simulink model "exampleModel_bus_axi_w_4ptavg"  (R2017b)
settings: Solver=VariableStepAuto  StartTime=0.0  StopTime=10e-5  RelTol=1e-3
PreLoadFcn:
  | setup
values from neighbouring files (symbols this model uses):
  axiClk = 156.25e6    (= 156250000)    [setup.m]    (also in setup_exampleModel_bus_axi_simulink.m; setup_exampleModel_bus_axi_simulink_lcls2.m; setup_lcls2_pcav.m; sysgen_signal.m)
  cav1p1_addr = 204    [setup_exampleModel_bus_axi_simulink.m]    (also in setup_exampleModel_bus_axi_simulink_lcls2.m; setup_lcls2_pcav.m; sysgen_signal.m)
  cav1p2_addr = cav1p1_addr * 2    (= 408)    [setup_exampleModel_bus_axi_simulink.m]    (also in setup_exampleModel_bus_axi_simulink_lcls2.m; setup_lcls2_pcav.m; sysgen_signal.m)
  cav2p1_addr = cav1p1_addr * 3    (= 612)    [setup_exampleModel_bus_axi_simulink.m]    (also in setup_exampleModel_bus_axi_simulink_lcls2.m; setup_lcls2_pcav.m; sysgen_signal.m)
  cav2p2_addr = cav1p1_addr * 4    (= 816)    [setup_exampleModel_bus_axi_simulink.m]    (also in setup_exampleModel_bus_axi_simulink_lcls2.m; setup_lcls2_pcav.m; sysgen_signal.m)
  Fadc = Fs/interleavedChannels    (= 29750000)    [setup.m]    (also in setup_exampleModel_bus_axi_simulink.m = 357000000; setup_exampleModel_bus_axi_simulink_lcls2.m = 351000000; setup_lcls2_pcav.m = 357000000; sysgen_signal.m = 357000000)
  fir_lpf = fir1(15, w_lpf)    [setup_exampleModel_bus_axi_simulink.m]    (also in setup_exampleModel_bus_axi_simulink_lcls2.m; setup_lcls2_pcav.m)
  Fproc = 204e6    (= 204000000)    [setup_exampleModel_bus_axi_simulink.m]    (also in setup_exampleModel_bus_axi_simulink_lcls2.m = 200571400; setup_lcls2_pcav.m; sysgen_signal.m)
  Fsig = Fproc/12    (= 17000000)    [setup_exampleModel_bus_axi_simulink.m]    (also in setup_exampleModel_bus_axi_simulink_lcls2.m = 16714283.3333; setup_lcls2_pcav.m)
  Tadc = 1/fadc    (= 2.80112044818e-09)    [cavity_signal.m]    (also in setup_exampleModel_bus_axi_simulink.m; setup_exampleModel_bus_axi_simulink_lcls2.m = 2.849002849e-09; setup_lcls2_pcav.m; setup_pcav_simulink.m)
undefined symbols (not defined in the file or in its folder): AXI4, Lite
libraries: xbsIndex_r4 x2870, llrf_lib x10, simulink x3
(part 14 of 15)

== system exampleModel_bus_axi_w_4ptavg/example/dsp/Cav2/Subsystem2/freq_err1/delta_phi ==
  note: 3.14
  note: calculating delta phi
  note: d(scaled_phi)
  phase : Inport
  window : Inport  Port=2
  reset : Inport  Port=3
  AddSub3 : xbsIndex_r4/AddSub  mode=Subtraction  use_carryin=off  use_carryout=off  en=on  latency=1  precision=Full  arith_type="Signed  (2's comp)"  n_bits=32  bin_pt=30  quantization=Truncate  overflow=Saturate  use_behavioral_HDL=off  hw_selection=Fabric  pipelined=off  dbl_ovrd=off  block_type=addsub
  Constant : xbsIndex_r4/Constant  const=0  gui_display_data_type=Fixed-point  arith_type=Signed (2's comp)  n_bits=1  bin_pt=0  preci_type=Single  exp_width=8  frac_width=24  explicit_period=off  period=1  equ=P=C  opselect=C  inp2=PCIN>>17  opr=+  inp1=P  carry=CIN  dbl_ovrd=off  block_type=constant
  Constant1 : xbsIndex_r4/Constant  const=0  gui_display_data_type=Fixed-point  arith_type=Signed (2's comp)  n_bits=1  bin_pt=0  preci_type=Single  exp_width=8  frac_width=24  explicit_period=off  period=1  equ=P=C  opselect=C  inp2=PCIN>>17  opr=+  inp1=P  carry=CIN  dbl_ovrd=off  block_type=constant
  Constant4 : xbsIndex_r4/Constant  const=pi  gui_display_data_type=Fixed-point  arith_type=Signed (2's comp)  n_bits=18  bin_pt=15  preci_type=Single  exp_width=8  frac_width=24  explicit_period=off  period=1  equ=P=C  opselect=C  inp2=PCIN>>17  opr=+  inp1=P  carry=CIN  dbl_ovrd=off  block_type=constant
  Convert1 : xbsIndex_r4/Convert  gui_display_data_type=Boolean  arith_type=Boolean  n_bits=16  bin_pt=14  float_type=Single  exp_bits=8  fraction_bits=24  quantization=Truncate  overflow=Wrap  en=off  latency=1  pipeline=off  dbl_ovrd=off  block_type=convert
  Delay2 : xbsIndex_r4/Delay  rst=off  infoeditControl=Selection of Reset will increase slice count due to use of real FFs and instead of SRLs  en=off  latency=2  reg_retiming=off  dbl_ovrd=off  block_type=delay
  Display{,1..2,5} (4 alike) : Display
  Gateway Out{3,27..29} (4 alike) : xbsIndex_r4/Gateway Out  inherit_from_input=off  hdl_port=on  rows=1  columns=1  UseAsDAC=off  DACChannel='1'  interface=None  automatic_assignment=on  address_offset=hex2dec('00')  intf_name=''  intf_description=''  timing_constraint=None  locs_specified=off  LOCs={}  io_standard={}  block_type=gatewayout
  Inverter : xbsIndex_r4/Inverter  en=off  latency=1  dbl_ovrd=off  block_type=inv
  Logical : xbsIndex_r4/Logical  logical_function=AND  inputs=2  en=off  latency=1  precision=User Defined  arith_type=Boolean  n_bits=1  bin_pt=0  align_bp=on  dbl_ovrd=off  block_type=logical
  Mult1 : xbsIndex_r4/Mult  precision=User Defined  arith_type="Signed  (2's comp)"  n_bits=32  bin_pt=30  quantization=Truncate  overflow=Saturate  en=off  latency=3  use_behavioral_HDL=off  opt=Speed  use_embedded=on  optimum_pipeline=off  pipeline=on  dbl_ovrd=off  use_rpm=on  placement_style=Triangular  block_type=mult
  Relational : xbsIndex_r4/Relational  mode=a!=b  op_type=Bool  en=off  latency=1  dbl_ovrd=off  block_type=relational
  Relational1 : xbsIndex_r4/Relational  mode=a!=b  op_type=Bool  en=off  latency=1  dbl_ovrd=off  block_type=relational
  low_bit : Scope  NumInputPorts=4
  phase_latching : Subsystem
  d_phi : Outport
  val_latched : Outport  Port=2
  wires:
  Logical/1 -> val_latched/1
  Relational1/1 -> Logical/2
  Relational/1 -> Logical/1
  phase_latching/2(Start_value) -> AddSub3/2, Gateway Out28/1, Relational1/1
  Constant1/1 -> Relational1/2
  Constant/1 -> Relational/2
  phase_latching/1(Stop_value) -> Gateway Out29/1, Relational/1, AddSub3/1
  window/1 -> phase_latching/2(window), Convert1/1
  Convert1/1 -> Inverter/1
  Gateway Out27/1 -> Display2/1, low_bit/3
  Gateway Out28/1 -> Display1/1, low_bit/2
  AddSub3/1 -> Gateway Out27/1, Mult1/1
  phase/1 -> phase_latching/1(phase)
  Mult1/1 -> Gateway Out3/1, d_phi/1
  Gateway Out29/1 -> Display/1, low_bit/1
  Delay2/1 -> AddSub3/3
  Gateway Out3/1 -> Display5/1, low_bit/4
  Constant4/1 -> Mult1/2
  Inverter/1 -> Delay2/1
  reset/1 -> phase_latching/3(reset)

== system exampleModel_bus_axi_w_4ptavg/example/dsp/Cav2/Subsystem2/freq_err1/delta_t ==
  note: (2*pi)/(Fsig)
  window : Inport
  reset : Inport  Port=2
  Constant5 : xbsIndex_r4/Constant  const=(2*pi)/(Fsig)  gui_display_data_type=Fixed-point  arith_type=Unsigned  n_bits=32  bin_pt=32  preci_type=Single  exp_width=8  frac_width=24  explicit_period=off  period=1  equ=P=C  opselect=C  inp2=PCIN>>17  opr=+  inp1=P  carry=CIN  dbl_ovrd=off  block_type=constant
  Convert1 : xbsIndex_r4/Convert  gui_display_data_type=Boolean  arith_type=Boolean  n_bits=16  bin_pt=14  float_type=Single  exp_bits=8  fraction_bits=24  quantization=Truncate  overflow=Wrap  en=off  latency=1  pipeline=off  dbl_ovrd=off  block_type=convert
  Counter2 : xbsIndex_r4/Counter  cnt_type=Free Running  cnt_to=Inf  operation=Up  start_count=0  cnt_by_val=1  arith_type=Unsigned  n_bits=10  bin_pt=0  load_pin=off  rst=on  en=on  explicit_period=on  period=1/(17e6)  use_behavioral_HDL=off  implementation=Fabric  dbl_ovrd=off  block_type=counter
  Display3 : Display
  Display4 : Display
  Gateway Out1 : xbsIndex_r4/Gateway Out  inherit_from_input=off  hdl_port=on  rows=1  columns=1  UseAsDAC=off  DACChannel='1'  interface=None  automatic_assignment=on  address_offset=hex2dec('00')  intf_name=''  intf_description=''  timing_constraint=None  locs_specified=off  LOCs={}  io_standard={}  block_type=gatewayout
  Gateway Out2 : xbsIndex_r4/Gateway Out  inherit_from_input=off  hdl_port=on  rows=1  columns=1  UseAsDAC=off  DACChannel='1'  interface=None  automatic_assignment=on  address_offset=hex2dec('00')  intf_name=''  intf_description=''  timing_constraint=None  locs_specified=off  LOCs={}  io_standard={}  block_type=gatewayout
  Inverter : xbsIndex_r4/Inverter  en=off  latency=1  dbl_ovrd=off  block_type=inv
  Mult : xbsIndex_r4/Mult  precision=User Defined  arith_type="Signed  (2's comp)"  n_bits=32  bin_pt=32  quantization=Truncate  overflow=Saturate  en=off  latency=3  use_behavioral_HDL=off  opt=Speed  use_embedded=on  optimum_pipeline=off  pipeline=on  dbl_ovrd=off  use_rpm=on  placement_style=Triangular  block_type=mult
  Register2 : xbsIndex_r4/Register  init=0  rst=on  en=on  dbl_ovrd=off  block_type=register
  dt : Outport
  wires:
  Gateway Out1/1 -> Display3/1
  window/1 -> Convert1/1
  Mult/1 -> Gateway Out1/1, dt/1
  Constant5/1 -> Mult/2
  Convert1/1 -> Counter2/2, Inverter/1
  Inverter/1 -> Register2/3
  Counter2/1 -> Register2/1
  Gateway Out2/1 -> Display4/1
  Register2/1 -> Gateway Out2/1, Mult/1
  reset/1 -> Counter2/1, Register2/2

== system exampleModel_bus_axi_w_4ptavg/example/dsp/Cav2/Subsystem4/freq_err1/Subsystem ==
  In1 : Inport
  In2 : Inport  Port=2
  AddSub : xbsIndex_r4/AddSub  mode=Addition  use_carryin=off  use_carryout=off  en=on  latency=1  precision=User Defined  arith_type="Signed  (2's comp)"  n_bits=64  bin_pt=32  quantization=Truncate  overflow=Saturate  use_behavioral_HDL=off  hw_selection=Fabric  pipelined=off  dbl_ovrd=off  block_type=addsub
  Constant1 : xbsIndex_r4/Constant  const=-Fsig  gui_display_data_type=Fixed-point  arith_type=Signed (2's comp)  n_bits=26  bin_pt=0  preci_type=Single  exp_width=8  frac_width=24  explicit_period=off  period=1  equ=P=C  opselect=C  inp2=PCIN>>17  opr=+  inp1=P  carry=CIN  dbl_ovrd=off  block_type=constant
  Convert1 : xbsIndex_r4/Convert  gui_display_data_type=Fixed-point  arith_type="Signed  (2's comp)"  n_bits=32  bin_pt=32  float_type=Single  exp_bits=8  fraction_bits=24  quantization=Truncate  overflow=Saturate  en=off  latency=1  pipeline=off  dbl_ovrd=off  block_type=convert
  Delay3 : xbsIndex_r4/Delay  rst=off  infoeditControl=Selection of Reset will increase slice count due to use of real FFs and instead of SRLs  en=off  latency=10  reg_retiming=off  dbl_ovrd=off  block_type=delay
  Delay4 : xbsIndex_r4/Delay  rst=off  infoeditControl=Selection of Reset will increase slice count due to use of real FFs and instead of SRLs  en=off  latency=1  reg_retiming=off  dbl_ovrd=off  block_type=delay
  Delay5 : xbsIndex_r4/Delay  rst=off  infoeditControl=Selection of Reset will increase slice count due to use of real FFs and instead of SRLs  en=off  latency=1  reg_retiming=off  dbl_ovrd=off  block_type=delay
  Display1 : Display
  Divide2 : xbsIndex_r4/Divide  flow_control=NonBlocking  axi_optimize_goal=Resources  algorithm_type=Radix2  infoedit1=Specify output fraction-width for Fixed-point division.  fractional_width=33  infoedit2=Specify latency for Floating-point division.  latency=1  rate=1  has_a_tlast=off  has_a_tuser=off  has_b_tlast=off  has_b_tuser=off  en=off  has_result_tready=off  result_tlast_behv=Pass_A_TLAST  has_underflow=off  has_overflow=off  has_invalid_op=off  has_divide_by_zero=off  fpo_op_type=mergeddivide  block_type=divide
      settings: infoedit=Blocking: Wait for data on all inputs, allow back-pressure.<br>NonBlocking: operate every cycle in which all inputs are valid, no back-pressure.
  Down Sample1 : xbsIndex_r4/Down Sample  sample_ratio=12  sample_phase="Last Value of Frame  (most efficient)"  en=off  rst=off  latency=1  dbl_ovrd=off  block_type=dsamp
  Down Sample8 : xbsIndex_r4/Down Sample  sample_ratio=12  sample_phase="Last Value of Frame  (most efficient)"  en=off  rst=off  latency=1  dbl_ovrd=off  block_type=dsamp
  Gateway Out{5..7,9} (4 alike) : xbsIndex_r4/Gateway Out  inherit_from_input=off  hdl_port=on  rows=1  columns=1  UseAsDAC=off  DACChannel='1'  interface=None  automatic_assignment=on  address_offset=hex2dec('00')  intf_name=''  intf_description=''  timing_constraint=None  locs_specified=off  LOCs={}  io_standard={}  block_type=gatewayout
  Inverter : xbsIndex_r4/Inverter  en=off  latency=1  dbl_ovrd=off  block_type=inv
  Logical1 : xbsIndex_r4/Logical  logical_function=AND  inputs=2  en=off  latency=1  precision=User Defined  arith_type=Boolean  n_bits=1  bin_pt=0  align_bp=on  dbl_ovrd=off  block_type=logical
  Register : xbsIndex_r4/Register  init=0  rst=on  en=on  dbl_ovrd=off  block_type=register
  Scope3 : Scope  NumInputPorts=3
  Scope4 : Scope  NumInputPorts=3
  tag scope: testb=global
  wires:
  Delay3/1 -> Logical1/2, Inverter/1
  Logical1/1 -> Gateway Out6/1, Delay4/1, Delay5/1, Register/3
  Constant1/1 -> Divide2/2
  Inverter/1 -> Logical1/1
  Divide2/1 -> Down Sample1/1
  Register/1 -> AddSub/1, Gateway Out5/1
  Gateway Out5/1 -> Scope3/2
  In2/1 -> Down Sample8/1
  Convert1/1 -> [testb]
  Down Sample8/1 -> Register/1
  Delay5/1 -> Register/2
  Delay4/1 -> AddSub/3
  Gateway Out6/1 -> Scope3/3
  In1/1 -> Delay3/1
  AddSub/1 -> AddSub/2, Gateway Out7/1, Divide2/1, Gateway Out9/1
  Down Sample1/1 -> Convert1/1
  Gateway Out7/1 -> Scope3/1, Display1/1
  Gateway Out9/1 -> Scope4/1

== system exampleModel_bus_axi_w_4ptavg/example/dsp/Cav2/Subsystem4/freq_err1/delta_phi ==
  note: 3.14
  note: calculating delta phi
  note: d(scaled_phi)
  phase : Inport
  window : Inport  Port=2
  reset : Inport  Port=3
  AddSub3 : xbsIndex_r4/AddSub  mode=Subtraction  use_carryin=off  use_carryout=off  en=on  latency=1  precision=Full  arith_type="Signed  (2's comp)"  n_bits=32  bin_pt=30  quantization=Truncate  overflow=Saturate  use_behavioral_HDL=off  hw_selection=Fabric  pipelined=off  dbl_ovrd=off  block_type=addsub
  Constant : xbsIndex_r4/Constant  const=0  gui_display_data_type=Fixed-point  arith_type=Signed (2's comp)  n_bits=1  bin_pt=0  preci_type=Single  exp_width=8  frac_width=24  explicit_period=off  period=1  equ=P=C  opselect=C  inp2=PCIN>>17  opr=+  inp1=P  carry=CIN  dbl_ovrd=off  block_type=constant
  Constant1 : xbsIndex_r4/Constant  const=0  gui_display_data_type=Fixed-point  arith_type=Signed (2's comp)  n_bits=1  bin_pt=0  preci_type=Single  exp_width=8  frac_width=24  explicit_period=off  period=1  equ=P=C  opselect=C  inp2=PCIN>>17  opr=+  inp1=P  carry=CIN  dbl_ovrd=off  block_type=constant
  Constant4 : xbsIndex_r4/Constant  const=pi  gui_display_data_type=Fixed-point  arith_type=Signed (2's comp)  n_bits=18  bin_pt=15  preci_type=Single  exp_width=8  frac_width=24  explicit_period=off  period=1  equ=P=C  opselect=C  inp2=PCIN>>17  opr=+  inp1=P  carry=CIN  dbl_ovrd=off  block_type=constant
  Convert1 : xbsIndex_r4/Convert  gui_display_data_type=Boolean  arith_type=Boolean  n_bits=16  bin_pt=14  float_type=Single  exp_bits=8  fraction_bits=24  quantization=Truncate  overflow=Wrap  en=off  latency=1  pipeline=off  dbl_ovrd=off  block_type=convert
  Delay2 : xbsIndex_r4/Delay  rst=off  infoeditControl=Selection of Reset will increase slice count due to use of real FFs and instead of SRLs  en=off  latency=2  reg_retiming=off  dbl_ovrd=off  block_type=delay
  Display{,1..2,5} (4 alike) : Display
  Gateway Out{3,27..29} (4 alike) : xbsIndex_r4/Gateway Out  inherit_from_input=off  hdl_port=on  rows=1  columns=1  UseAsDAC=off  DACChannel='1'  interface=None  automatic_assignment=on  address_offset=hex2dec('00')  intf_name=''  intf_description=''  timing_constraint=None  locs_specified=off  LOCs={}  io_standard={}  block_type=gatewayout
  Inverter : xbsIndex_r4/Inverter  en=off  latency=1  dbl_ovrd=off  block_type=inv
  Logical : xbsIndex_r4/Logical  logical_function=AND  inputs=2  en=off  latency=1  precision=User Defined  arith_type=Boolean  n_bits=1  bin_pt=0  align_bp=on  dbl_ovrd=off  block_type=logical
  Mult1 : xbsIndex_r4/Mult  precision=User Defined  arith_type="Signed  (2's comp)"  n_bits=32  bin_pt=30  quantization=Truncate  overflow=Saturate  en=off  latency=3  use_behavioral_HDL=off  opt=Speed  use_embedded=on  optimum_pipeline=off  pipeline=on  dbl_ovrd=off  use_rpm=on  placement_style=Triangular  block_type=mult
  Relational : xbsIndex_r4/Relational  mode=a!=b  op_type=Bool  en=off  latency=1  dbl_ovrd=off  block_type=relational
  Relational1 : xbsIndex_r4/Relational  mode=a!=b  op_type=Bool  en=off  latency=1  dbl_ovrd=off  block_type=relational
  low_bit : Scope  NumInputPorts=4
  phase_latching : Subsystem
  d_phi : Outport
  val_latched : Outport  Port=2
  wires:
  Logical/1 -> val_latched/1
  Relational1/1 -> Logical/2
  Relational/1 -> Logical/1
  phase_latching/2(Start_value) -> AddSub3/2, Gateway Out28/1, Relational1/1
  Constant1/1 -> Relational1/2
  Constant/1 -> Relational/2
  phase_latching/1(Stop_value) -> Gateway Out29/1, Relational/1, AddSub3/1
  window/1 -> phase_latching/2(window), Convert1/1
  Convert1/1 -> Inverter/1
  Gateway Out27/1 -> Display2/1, low_bit/3
  Gateway Out28/1 -> Display1/1, low_bit/2
  AddSub3/1 -> Gateway Out27/1, Mult1/1
  phase/1 -> phase_latching/1(phase)
  Mult1/1 -> Gateway Out3/1, d_phi/1
  Gateway Out29/1 -> Display/1, low_bit/1
  Delay2/1 -> AddSub3/3
  Gateway Out3/1 -> Display5/1, low_bit/4
  Constant4/1 -> Mult1/2
  Inverter/1 -> Delay2/1
  reset/1 -> phase_latching/3(reset)

== system exampleModel_bus_axi_w_4ptavg/example/dsp/Cav2/Subsystem4/freq_err1/delta_t ==
  note: (2*pi)/(Fsig)
  window : Inport
  reset : Inport  Port=2
  Constant5 : xbsIndex_r4/Constant  const=(2*pi)/(Fsig)  gui_display_data_type=Fixed-point  arith_type=Unsigned  n_bits=32  bin_pt=32  preci_type=Single  exp_width=8  frac_width=24  explicit_period=off  period=1  equ=P=C  opselect=C  inp2=PCIN>>17  opr=+  inp1=P  carry=CIN  dbl_ovrd=off  block_type=constant
  Convert1 : xbsIndex_r4/Convert  gui_display_data_type=Boolean  arith_type=Boolean  n_bits=16  bin_pt=14  float_type=Single  exp_bits=8  fraction_bits=24  quantization=Truncate  overflow=Wrap  en=off  latency=1  pipeline=off  dbl_ovrd=off  block_type=convert
  Counter2 : xbsIndex_r4/Counter  cnt_type=Free Running  cnt_to=Inf  operation=Up  start_count=0  cnt_by_val=1  arith_type=Unsigned  n_bits=10  bin_pt=0  load_pin=off  rst=on  en=on  explicit_period=on  period=1/(17e6)  use_behavioral_HDL=off  implementation=Fabric  dbl_ovrd=off  block_type=counter
  Display3 : Display
  Display4 : Display
  Gateway Out1 : xbsIndex_r4/Gateway Out  inherit_from_input=off  hdl_port=on  rows=1  columns=1  UseAsDAC=off  DACChannel='1'  interface=None  automatic_assignment=on  address_offset=hex2dec('00')  intf_name=''  intf_description=''  timing_constraint=None  locs_specified=off  LOCs={}  io_standard={}  block_type=gatewayout
  Gateway Out2 : xbsIndex_r4/Gateway Out  inherit_from_input=off  hdl_port=on  rows=1  columns=1  UseAsDAC=off  DACChannel='1'  interface=None  automatic_assignment=on  address_offset=hex2dec('00')  intf_name=''  intf_description=''  timing_constraint=None  locs_specified=off  LOCs={}  io_standard={}  block_type=gatewayout
  Inverter : xbsIndex_r4/Inverter  en=off  latency=1  dbl_ovrd=off  block_type=inv
  Mult : xbsIndex_r4/Mult  precision=User Defined  arith_type="Signed  (2's comp)"  n_bits=32  bin_pt=32  quantization=Truncate  overflow=Saturate  en=off  latency=3  use_behavioral_HDL=off  opt=Speed  use_embedded=on  optimum_pipeline=off  pipeline=on  dbl_ovrd=off  use_rpm=on  placement_style=Triangular  block_type=mult
  Register2 : xbsIndex_r4/Register  init=0  rst=on  en=on  dbl_ovrd=off  block_type=register
  dt : Outport
  wires:
  Gateway Out1/1 -> Display3/1
  window/1 -> Convert1/1
  Mult/1 -> Gateway Out1/1, dt/1
  Constant5/1 -> Mult/2
  Convert1/1 -> Counter2/2, Inverter/1
  Inverter/1 -> Register2/3
  Counter2/1 -> Register2/1
  Gateway Out2/1 -> Display4/1
  Register2/1 -> Gateway Out2/1, Mult/1
  reset/1 -> Counter2/1, Register2/2

== system exampleModel_bus_axi_w_4ptavg/example/dsp/Cav2/c2p1_window_wf /Delay_calc1/Subsystem ==
  In1 : Inport
  Delay3 : xbsIndex_r4/Delay  rst=off  infoeditControl=Selection of Reset will increase slice count due to use of real FFs and instead of SRLs  en=off  latency=2  reg_retiming=off  dbl_ovrd=off  block_type=delay
  Inverter5 : xbsIndex_r4/Inverter  en=off  latency=1  dbl_ovrd=off  block_type=inv
  Logical1 : xbsIndex_r4/Logical  logical_function=AND  inputs=2  en=off  latency=1  precision=Full  arith_type=Unsigned  n_bits=16  bin_pt=0  align_bp=on  dbl_ovrd=off  block_type=logical
  Out1 : Outport
  wires:
  In1/1 -> Inverter5/1, Delay3/1
  Inverter5/1 -> Logical1/1
  Logical1/1 -> Out1/1
  Delay3/1 -> Logical1/2

== system exampleModel_bus_axi_w_4ptavg/example/dsp/Cav2/c2p1_window_wf /Delay_calc1/Subsystem1 ==
  lc : Inport
  d : Inport  Port=2
  qb : Inport  Port=3
  Inverter1 : xbsIndex_r4/Inverter  en=off  latency=1  dbl_ovrd=off  block_type=inv
  Logical6 : xbsIndex_r4/Logical  logical_function=OR  inputs=2  en=off  latency=1  precision=Full  arith_type=Unsigned  n_bits=16  bin_pt=0  align_bp=on  dbl_ovrd=off  block_type=logical
  Register1 : xbsIndex_r4/Register  init=0  rst=off  en=on  dbl_ovrd=off  block_type=register
  q : Outport
  wires:
  qb/1 -> Inverter1/1
  d/1 -> Register1/1
  Logical6/1 -> Register1/2
  lc/1 -> Logical6/2
  Register1/1 -> q/1
  Inverter1/1 -> Logical6/1

== system exampleModel_bus_axi_w_4ptavg/example/dsp/Cav2/c2p1_window_wf /Delay_calc1/Subsystem2 ==
  lc : Inport
  d : Inport  Port=2
  qb : Inport  Port=3
  Inverter1 : xbsIndex_r4/Inverter  en=off  latency=1  dbl_ovrd=off  block_type=inv
  Logical6 : xbsIndex_r4/Logical  logical_function=OR  inputs=2  en=off  latency=1  precision=Full  arith_type=Unsigned  n_bits=16  bin_pt=0  align_bp=on  dbl_ovrd=off  block_type=logical
  Register1 : xbsIndex_r4/Register  init=0  rst=off  en=on  dbl_ovrd=off  block_type=register
  q : Outport
  wires:
  Inverter1/1 -> Logical6/1
  Register1/1 -> q/1
  lc/1 -> Logical6/2
  Logical6/1 -> Register1/2
  d/1 -> Register1/1
  qb/1 -> Inverter1/1

== system exampleModel_bus_axi_w_4ptavg/example/dsp/Cav2/c2p1_window_wf /Delay_calc1/Subsystem3 ==
  In1 : Inport
  In2 : Inport  Port=2
  Gateway Out{1..2,18..19} (4 alike) : xbsIndex_r4/Gateway Out  inherit_from_input=off  hdl_port=off  rows=1  columns=1  UseAsDAC=off  DACChannel='1'  interface=None  automatic_assignment=on  address_offset=hex2dec('00')  intf_name=''  intf_description=''  timing_constraint=None  locs_specified=off  LOCs={}  io_standard={}  block_type=gatewayout
  Logical2 : xbsIndex_r4/Logical  logical_function=AND  inputs=2  en=off  latency=1  precision=Full  arith_type=Unsigned  n_bits=16  bin_pt=0  align_bp=on  dbl_ovrd=off  block_type=logical
  Logical7 : xbsIndex_r4/Logical  logical_function=OR  inputs=2  en=off  latency=1  precision=Full  arith_type=Unsigned  n_bits=16  bin_pt=0  align_bp=on  dbl_ovrd=off  block_type=logical
  Scope1 : Scope  NumInputPorts=2
  Scope3 : Scope  NumInputPorts=2
  and : Outport
  or : Outport  Port=2
  wires:
  In1/1 -> Gateway Out18/1, Logical7/1, Logical2/1
  Logical7/1 -> Gateway Out2/1, or/1
  In2/1 -> Gateway Out19/1, Logical2/2, Logical7/2
  Logical2/1 -> Gateway Out1/1, and/1
  Gateway Out19/1 -> Scope3/2
  Gateway Out18/1 -> Scope3/1
  Gateway Out1/1 -> Scope1/1
  Gateway Out2/1 -> Scope1/2

== system exampleModel_bus_axi_w_4ptavg/example/dsp/Cav2/c2p1_window_wf /Delay_calc1/negedge ==
  d : Inport
  Delay1 : xbsIndex_r4/Delay  rst=off  infoeditControl=Selection of Reset will increase slice count due to use of real FFs and instead of SRLs  en=off  latency=4  reg_retiming=off  dbl_ovrd=off  block_type=delay
  Delay2 : xbsIndex_r4/Delay  rst=off  infoeditControl=Selection of Reset will increase slice count due to use of real FFs and instead of SRLs  en=off  latency=20  reg_retiming=off  dbl_ovrd=off  block_type=delay
  Inverter4 : xbsIndex_r4/Inverter  en=off  latency=1  dbl_ovrd=off  block_type=inv
  Logical7 : xbsIndex_r4/Logical  logical_function=AND  inputs=2  en=off  latency=1  precision=Full  arith_type=Unsigned  n_bits=16  bin_pt=0  align_bp=on  dbl_ovrd=off  block_type=logical
  q : Outport
  wires:
  Delay1/1 -> Logical7/2
  d/1 -> Delay2/1
  Inverter4/1 -> Logical7/1
  Logical7/1 -> q/1
  Delay2/1 -> Inverter4/1, Delay1/1

== system exampleModel_bus_axi_w_4ptavg/example/dsp/Cav2/c2p1_window_wf /Delay_calc2/Subsystem ==
  In1 : Inport
  Delay3 : xbsIndex_r4/Delay  rst=off  infoeditControl=Selection of Reset will increase slice count due to use of real FFs and instead of SRLs  en=off  latency=2  reg_retiming=off  dbl_ovrd=off  block_type=delay
  Inverter5 : xbsIndex_r4/Inverter  en=off  latency=1  dbl_ovrd=off  block_type=inv
  Logical1 : xbsIndex_r4/Logical  logical_function=AND  inputs=2  en=off  latency=1  precision=Full  arith_type=Unsigned  n_bits=16  bin_pt=0  align_bp=on  dbl_ovrd=off  block_type=logical
  Out1 : Outport
  wires:
  In1/1 -> Inverter5/1, Delay3/1
  Inverter5/1 -> Logical1/1
  Logical1/1 -> Out1/1
  Delay3/1 -> Logical1/2

== system exampleModel_bus_axi_w_4ptavg/example/dsp/Cav2/c2p1_window_wf /Delay_calc2/Subsystem1 ==
  lc : Inport
  d : Inport  Port=2
  qb : Inport  Port=3
  Inverter1 : xbsIndex_r4/Inverter  en=off  latency=1  dbl_ovrd=off  block_type=inv
  Logical6 : xbsIndex_r4/Logical  logical_function=OR  inputs=2  en=off  latency=1  precision=Full  arith_type=Unsigned  n_bits=16  bin_pt=0  align_bp=on  dbl_ovrd=off  block_type=logical
  Register1 : xbsIndex_r4/Register  init=0  rst=off  en=on  dbl_ovrd=off  block_type=register
  q : Outport
  wires:
  qb/1 -> Inverter1/1
  d/1 -> Register1/1
  Logical6/1 -> Register1/2
  lc/1 -> Logical6/2
  Register1/1 -> q/1
  Inverter1/1 -> Logical6/1

== system exampleModel_bus_axi_w_4ptavg/example/dsp/Cav2/c2p1_window_wf /Delay_calc2/Subsystem2 ==
  lc : Inport
  d : Inport  Port=2
  qb : Inport  Port=3
  Inverter1 : xbsIndex_r4/Inverter  en=off  latency=1  dbl_ovrd=off  block_type=inv
  Logical6 : xbsIndex_r4/Logical  logical_function=OR  inputs=2  en=off  latency=1  precision=Full  arith_type=Unsigned  n_bits=16  bin_pt=0  align_bp=on  dbl_ovrd=off  block_type=logical
  Register1 : xbsIndex_r4/Register  init=0  rst=off  en=on  dbl_ovrd=off  block_type=register
  q : Outport
  wires:
  Inverter1/1 -> Logical6/1
  Register1/1 -> q/1
  lc/1 -> Logical6/2
  Logical6/1 -> Register1/2
  d/1 -> Register1/1
  qb/1 -> Inverter1/1

== system exampleModel_bus_axi_w_4ptavg/example/dsp/Cav2/c2p1_window_wf /Delay_calc2/Subsystem3 ==
  In1 : Inport
  In2 : Inport  Port=2
  Gateway Out{1..2,18..19} (4 alike) : xbsIndex_r4/Gateway Out  inherit_from_input=off  hdl_port=off  rows=1  columns=1  UseAsDAC=off  DACChannel='1'  interface=None  automatic_assignment=on  address_offset=hex2dec('00')  intf_name=''  intf_description=''  timing_constraint=None  locs_specified=off  LOCs={}  io_standard={}  block_type=gatewayout
  Logical2 : xbsIndex_r4/Logical  logical_function=AND  inputs=2  en=off  latency=1  precision=Full  arith_type=Unsigned  n_bits=16  bin_pt=0  align_bp=on  dbl_ovrd=off  block_type=logical
  Logical7 : xbsIndex_r4/Logical  logical_function=OR  inputs=2  en=off  latency=1  precision=Full  arith_type=Unsigned  n_bits=16  bin_pt=0  align_bp=on  dbl_ovrd=off  block_type=logical
  Scope1 : Scope  NumInputPorts=2
  Scope3 : Scope  NumInputPorts=2
  and : Outport
  or : Outport  Port=2
  wires:
  In1/1 -> Gateway Out18/1, Logical7/1, Logical2/1
  Logical7/1 -> Gateway Out2/1, or/1
  In2/1 -> Gateway Out19/1, Logical2/2, Logical7/2
  Logical2/1 -> Gateway Out1/1, and/1
  Gateway Out19/1 -> Scope3/2
  Gateway Out18/1 -> Scope3/1
  Gateway Out1/1 -> Scope1/1
  Gateway Out2/1 -> Scope1/2

== system exampleModel_bus_axi_w_4ptavg/example/dsp/Cav2/c2p1_window_wf /Delay_calc2/negedge ==
  d : Inport
  Delay1 : xbsIndex_r4/Delay  rst=off  infoeditControl=Selection of Reset will increase slice count due to use of real FFs and instead of SRLs  en=off  latency=4  reg_retiming=off  dbl_ovrd=off  block_type=delay
  Delay2 : xbsIndex_r4/Delay  rst=off  infoeditControl=Selection of Reset will increase slice count due to use of real FFs and instead of SRLs  en=off  latency=20  reg_retiming=off  dbl_ovrd=off  block_type=delay
  Inverter4 : xbsIndex_r4/Inverter  en=off  latency=1  dbl_ovrd=off  block_type=inv
  Logical7 : xbsIndex_r4/Logical  logical_function=AND  inputs=2  en=off  latency=1  precision=Full  arith_type=Unsigned  n_bits=16  bin_pt=0  align_bp=on  dbl_ovrd=off  block_type=logical
  q : Outport
  wires:
  Delay1/1 -> Logical7/2
  d/1 -> Delay2/1
  Inverter4/1 -> Logical7/1
  Logical7/1 -> q/1
  Delay2/1 -> Inverter4/1, Delay1/1

== system exampleModel_bus_axi_w_4ptavg/example/dsp/Cav2/c2p2_window_wf/Delay_calc1/Subsystem ==
  In1 : Inport
  Delay3 : xbsIndex_r4/Delay  rst=off  infoeditControl=Selection of Reset will increase slice count due to use of real FFs and instead of SRLs  en=off  latency=2  reg_retiming=off  dbl_ovrd=off  block_type=delay
  Inverter5 : xbsIndex_r4/Inverter  en=off  latency=1  dbl_ovrd=off  block_type=inv
  Logical1 : xbsIndex_r4/Logical  logical_function=AND  inputs=2  en=off  latency=1  precision=Full  arith_type=Unsigned  n_bits=16  bin_pt=0  align_bp=on  dbl_ovrd=off  block_type=logical
  Out1 : Outport
  wires:
  In1/1 -> Inverter5/1, Delay3/1
  Inverter5/1 -> Logical1/1
  Logical1/1 -> Out1/1
  Delay3/1 -> Logical1/2

== system exampleModel_bus_axi_w_4ptavg/example/dsp/Cav2/c2p2_window_wf/Delay_calc1/Subsystem1 ==
  lc : Inport
  d : Inport  Port=2
  qb : Inport  Port=3
  Inverter1 : xbsIndex_r4/Inverter  en=off  latency=1  dbl_ovrd=off  block_type=inv
  Logical6 : xbsIndex_r4/Logical  logical_function=OR  inputs=2  en=off  latency=1  precision=Full  arith_type=Unsigned  n_bits=16  bin_pt=0  align_bp=on  dbl_ovrd=off  block_type=logical
  Register1 : xbsIndex_r4/Register  init=0  rst=off  en=on  dbl_ovrd=off  block_type=register
  q : Outport
  wires:
  qb/1 -> Inverter1/1
  d/1 -> Register1/1
  Logical6/1 -> Register1/2
  lc/1 -> Logical6/2
  Register1/1 -> q/1
  Inverter1/1 -> Logical6/1

== system exampleModel_bus_axi_w_4ptavg/example/dsp/Cav2/c2p2_window_wf/Delay_calc1/Subsystem2 ==
  lc : Inport
  d : Inport  Port=2
  qb : Inport  Port=3
  Inverter1 : xbsIndex_r4/Inverter  en=off  latency=1  dbl_ovrd=off  block_type=inv
  Logical6 : xbsIndex_r4/Logical  logical_function=OR  inputs=2  en=off  latency=1  precision=Full  arith_type=Unsigned  n_bits=16  bin_pt=0  align_bp=on  dbl_ovrd=off  block_type=logical
  Register1 : xbsIndex_r4/Register  init=0  rst=off  en=on  dbl_ovrd=off  block_type=register
  q : Outport
  wires:
  Inverter1/1 -> Logical6/1
  Register1/1 -> q/1
  lc/1 -> Logical6/2
  Logical6/1 -> Register1/2
  d/1 -> Register1/1
  qb/1 -> Inverter1/1

== system exampleModel_bus_axi_w_4ptavg/example/dsp/Cav2/c2p2_window_wf/Delay_calc1/Subsystem3 ==
  In1 : Inport
  In2 : Inport  Port=2
  Gateway Out{1..2,18..19} (4 alike) : xbsIndex_r4/Gateway Out  inherit_from_input=off  hdl_port=off  rows=1  columns=1  UseAsDAC=off  DACChannel='1'  interface=None  automatic_assignment=on  address_offset=hex2dec('00')  intf_name=''  intf_description=''  timing_constraint=None  locs_specified=off  LOCs={}  io_standard={}  block_type=gatewayout
  Logical2 : xbsIndex_r4/Logical  logical_function=AND  inputs=2  en=off  latency=1  precision=Full  arith_type=Unsigned  n_bits=16  bin_pt=0  align_bp=on  dbl_ovrd=off  block_type=logical
  Logical7 : xbsIndex_r4/Logical  logical_function=OR  inputs=2  en=off  latency=1  precision=Full  arith_type=Unsigned  n_bits=16  bin_pt=0  align_bp=on  dbl_ovrd=off  block_type=logical
  Scope1 : Scope  NumInputPorts=2
  Scope3 : Scope  NumInputPorts=2
  and : Outport
  or : Outport  Port=2
  wires:
  In1/1 -> Gateway Out18/1, Logical7/1, Logical2/1
  Logical7/1 -> Gateway Out2/1, or/1
  In2/1 -> Gateway Out19/1, Logical2/2, Logical7/2
  Logical2/1 -> Gateway Out1/1, and/1
  Gateway Out19/1 -> Scope3/2
  Gateway Out18/1 -> Scope3/1
  Gateway Out1/1 -> Scope1/1
  Gateway Out2/1 -> Scope1/2

== system exampleModel_bus_axi_w_4ptavg/example/dsp/Cav2/c2p2_window_wf/Delay_calc1/negedge ==
  d : Inport
  Delay1 : xbsIndex_r4/Delay  rst=off  infoeditControl=Selection of Reset will increase slice count due to use of real FFs and instead of SRLs  en=off  latency=4  reg_retiming=off  dbl_ovrd=off  block_type=delay
  Delay2 : xbsIndex_r4/Delay  rst=off  infoeditControl=Selection of Reset will increase slice count due to use of real FFs and instead of SRLs  en=off  latency=20  reg_retiming=off  dbl_ovrd=off  block_type=delay
  Inverter4 : xbsIndex_r4/Inverter  en=off  latency=1  dbl_ovrd=off  block_type=inv
  Logical7 : xbsIndex_r4/Logical  logical_function=AND  inputs=2  en=off  latency=1  precision=Full  arith_type=Unsigned  n_bits=16  bin_pt=0  align_bp=on  dbl_ovrd=off  block_type=logical
  q : Outport
  wires:
  Delay1/1 -> Logical7/2
  d/1 -> Delay2/1
  Inverter4/1 -> Logical7/1
  Logical7/1 -> q/1
  Delay2/1 -> Inverter4/1, Delay1/1

== system exampleModel_bus_axi_w_4ptavg/example/dsp/Cav2/c2p2_window_wf/Delay_calc2/Subsystem ==
  In1 : Inport
  Delay3 : xbsIndex_r4/Delay  rst=off  infoeditControl=Selection of Reset will increase slice count due to use of real FFs and instead of SRLs  en=off  latency=2  reg_retiming=off  dbl_ovrd=off  block_type=delay
  Inverter5 : xbsIndex_r4/Inverter  en=off  latency=1  dbl_ovrd=off  block_type=inv
  Logical1 : xbsIndex_r4/Logical  logical_function=AND  inputs=2  en=off  latency=1  precision=Full  arith_type=Unsigned  n_bits=16  bin_pt=0  align_bp=on  dbl_ovrd=off  block_type=logical
  Out1 : Outport
  wires:
  Delay3/1 -> Logical1/2
  Logical1/1 -> Out1/1
  Inverter5/1 -> Logical1/1
  In1/1 -> Delay3/1, Inverter5/1

== system exampleModel_bus_axi_w_4ptavg/example/dsp/Cav2/c2p2_window_wf/Delay_calc2/Subsystem1 ==
  lc : Inport
  d : Inport  Port=2
  qb : Inport  Port=3
  Inverter1 : xbsIndex_r4/Inverter  en=off  latency=1  dbl_ovrd=off  block_type=inv
  Logical6 : xbsIndex_r4/Logical  logical_function=OR  inputs=2  en=off  latency=1  precision=Full  arith_type=Unsigned  n_bits=16  bin_pt=0  align_bp=on  dbl_ovrd=off  block_type=logical
  Register1 : xbsIndex_r4/Register  init=0  rst=off  en=on  dbl_ovrd=off  block_type=register
  q : Outport
  wires:
  Inverter1/1 -> Logical6/1
  Register1/1 -> q/1
  lc/1 -> Logical6/2
  Logical6/1 -> Register1/2
  d/1 -> Register1/1
  qb/1 -> Inverter1/1

== system exampleModel_bus_axi_w_4ptavg/example/dsp/Cav2/c2p2_window_wf/Delay_calc2/Subsystem2 ==
  lc : Inport
  d : Inport  Port=2
  qb : Inport  Port=3
  Inverter1 : xbsIndex_r4/Inverter  en=off  latency=1  dbl_ovrd=off  block_type=inv
  Logical6 : xbsIndex_r4/Logical  logical_function=OR  inputs=2  en=off  latency=1  precision=Full  arith_type=Unsigned  n_bits=16  bin_pt=0  align_bp=on  dbl_ovrd=off  block_type=logical
  Register1 : xbsIndex_r4/Register  init=0  rst=off  en=on  dbl_ovrd=off  block_type=register
  q : Outport
  wires:
  qb/1 -> Inverter1/1
  d/1 -> Register1/1
  Logical6/1 -> Register1/2
  lc/1 -> Logical6/2
  Register1/1 -> q/1
  Inverter1/1 -> Logical6/1

== system exampleModel_bus_axi_w_4ptavg/example/dsp/Cav2/c2p2_window_wf/Delay_calc2/Subsystem3 ==
  In1 : Inport
  In2 : Inport  Port=2
  Gateway Out{1..2,18..19} (4 alike) : xbsIndex_r4/Gateway Out  inherit_from_input=off  hdl_port=off  rows=1  columns=1  UseAsDAC=off  DACChannel='1'  interface=None  automatic_assignment=on  address_offset=hex2dec('00')  intf_name=''  intf_description=''  timing_constraint=None  locs_specified=off  LOCs={}  io_standard={}  block_type=gatewayout
  Logical2 : xbsIndex_r4/Logical  logical_function=AND  inputs=2  en=off  latency=1  precision=Full  arith_type=Unsigned  n_bits=16  bin_pt=0  align_bp=on  dbl_ovrd=off  block_type=logical
  Logical7 : xbsIndex_r4/Logical  logical_function=OR  inputs=2  en=off  latency=1  precision=Full  arith_type=Unsigned  n_bits=16  bin_pt=0  align_bp=on  dbl_ovrd=off  block_type=logical
  Scope1 : Scope  NumInputPorts=2
  Scope3 : Scope  NumInputPorts=2
  and : Outport
  or : Outport  Port=2
  wires:
  Gateway Out2/1 -> Scope1/2
  Gateway Out1/1 -> Scope1/1
  Gateway Out18/1 -> Scope3/1
  Gateway Out19/1 -> Scope3/2
  Logical2/1 -> and/1, Gateway Out1/1
  In2/1 -> Logical7/2, Logical2/2, Gateway Out19/1
  Logical7/1 -> or/1, Gateway Out2/1
  In1/1 -> Logical2/1, Logical7/1, Gateway Out18/1

== system exampleModel_bus_axi_w_4ptavg/example/dsp/Cav2/c2p2_window_wf/Delay_calc2/negedge ==
  d : Inport
  Delay1 : xbsIndex_r4/Delay  rst=off  infoeditControl=Selection of Reset will increase slice count due to use of real FFs and instead of SRLs  en=off  latency=4  reg_retiming=off  dbl_ovrd=off  block_type=delay
  Delay2 : xbsIndex_r4/Delay  rst=off  infoeditControl=Selection of Reset will increase slice count due to use of real FFs and instead of SRLs  en=off  latency=20  reg_retiming=off  dbl_ovrd=off  block_type=delay
  Inverter4 : xbsIndex_r4/Inverter  en=off  latency=1  dbl_ovrd=off  block_type=inv
  Logical7 : xbsIndex_r4/Logical  logical_function=AND  inputs=2  en=off  latency=1  precision=Full  arith_type=Unsigned  n_bits=16  bin_pt=0  align_bp=on  dbl_ovrd=off  block_type=logical
  q : Outport
  wires:
  Delay2/1 -> Delay1/1, Inverter4/1
  Logical7/1 -> q/1
  Inverter4/1 -> Logical7/1
  d/1 -> Delay2/1
  Delay1/1 -> Logical7/2

== system exampleModel_bus_axi_w_4ptavg/example/dsp/Cav1/Subsystem/freq_err/delta_phi/phase_latching ==
  phase : Inport
  window : Inport  Port=2
  reset : Inport  Port=3
  AddSub1 : xbsIndex_r4/AddSub  mode=Subtraction  use_carryin=off  use_carryout=off  en=off  latency=1  precision=User Defined  arith_type="Signed  (2's comp)"  n_bits=2  bin_pt=0  quantization=Truncate  overflow=Saturate  use_behavioral_HDL=off  hw_selection=Fabric  pipelined=off  dbl_ovrd=off  block_type=addsub
  AddSub2 : xbsIndex_r4/AddSub  mode=Subtraction  use_carryin=off  use_carryout=off  en=off  latency=1  precision=User Defined  arith_type="Signed  (2's comp)"  n_bits=2  bin_pt=0  quantization=Truncate  overflow=Saturate  use_behavioral_HDL=off  hw_selection=Fabric  pipelined=off  dbl_ovrd=off  block_type=addsub
  Constant2 : xbsIndex_r4/Constant  const=0  gui_display_data_type=Fixed-point  arith_type=Signed (2's comp)  n_bits=1  bin_pt=0  preci_type=Single  exp_width=8  frac_width=24  explicit_period=off  period=1  equ=P=C  opselect=C  inp2=PCIN>>17  opr=+  inp1=P  carry=CIN  dbl_ovrd=off  block_type=constant
  Constant3 : xbsIndex_r4/Constant  const=0  gui_display_data_type=Fixed-point  arith_type=Signed (2's comp)  n_bits=1  bin_pt=0  preci_type=Single  exp_width=8  frac_width=24  explicit_period=off  period=1  equ=P=C  opselect=C  inp2=PCIN>>17  opr=+  inp1=P  carry=CIN  dbl_ovrd=off  block_type=constant
  Delay4 : xbsIndex_r4/Delay  rst=off  infoeditControl=Selection of Reset will increase slice count due to use of real FFs and instead of SRLs  en=off  latency=1  reg_retiming=off  dbl_ovrd=off  block_type=delay
  Delay5 : xbsIndex_r4/Delay  rst=off  infoeditControl=Selection of Reset will increase slice count due to use of real FFs and instead of SRLs  en=off  latency=1  reg_retiming=off  dbl_ovrd=off  block_type=delay
  Delay6 : xbsIndex_r4/Delay  rst=off  infoeditControl=Selection of Reset will increase slice count due to use of real FFs and instead of SRLs  en=off  latency=1  reg_retiming=off  dbl_ovrd=off  block_type=delay
  Gateway Out{,1..5} (6 alike) : xbsIndex_r4/Gateway Out  inherit_from_input=off  hdl_port=on  rows=1  columns=1  UseAsDAC=off  DACChannel='1'  interface=None  automatic_assignment=on  address_offset=hex2dec('00')  intf_name=''  intf_description=''  timing_constraint=None  locs_specified=off  LOCs={}  io_standard={}  block_type=gatewayout
  Register : xbsIndex_r4/Register  init=0  rst=on  en=on  dbl_ovrd=off  block_type=register
  Register1 : xbsIndex_r4/Register  init=0  rst=on  en=on  dbl_ovrd=off  block_type=register
  Relational : xbsIndex_r4/Relational  mode=a>b  op_type=Bool  en=off  latency=1  dbl_ovrd=off  block_type=relational
  Relational1 : xbsIndex_r4/Relational  mode=a>b  op_type=Bool  en=off  latency=1  dbl_ovrd=off  block_type=relational
  Scope1 : Scope  NumInputPorts=3
  Scope3 : Scope  NumInputPorts=3
  Stop_value : Outport
  Start_value : Outport  Port=2
  wires:
  Register/1 -> Gateway Out3/1, Start_value/1
  Constant3/1 -> Relational1/2
  AddSub2/1 -> Relational1/1
  Constant2/1 -> Relational/2
  Delay6/1 -> AddSub2/1
  Delay4/1 -> AddSub1/2
  phase/1 -> Register1/1, Gateway Out/1, Register/1
  AddSub1/1 -> Relational/1
  Delay5/1 -> Gateway Out2/1, Register/3
  Relational1/1 -> Gateway Out1/1, Register1/3
  Register1/1 -> Gateway Out4/1, Stop_value/1
  Relational/1 -> Delay5/1
  window/1 -> AddSub1/1, Delay4/1, AddSub2/2, Delay6/1
  reset/1 -> Gateway Out5/1, Register1/2, Register/2
  Gateway Out/1 -> Scope3/1
  Gateway Out1/1 -> Scope3/2
  Gateway Out2/1 -> Scope3/3
  Gateway Out5/1 -> Scope1/3
  Gateway Out4/1 -> Scope1/2
  Gateway Out3/1 -> Scope1/1

== system exampleModel_bus_axi_w_4ptavg/example/dsp/Cav1/c1p1_freq_err_module/freq_err1/delta_phi/phase_latching ==
  phase : Inport
  window : Inport  Port=2
  reset : Inport  Port=3
  AddSub1 : xbsIndex_r4/AddSub  mode=Subtraction  use_carryin=off  use_carryout=off  en=off  latency=1  precision=User Defined  arith_type="Signed  (2's comp)"  n_bits=2  bin_pt=0  quantization=Truncate  overflow=Saturate  use_behavioral_HDL=off  hw_selection=Fabric  pipelined=off  dbl_ovrd=off  block_type=addsub
  AddSub2 : xbsIndex_r4/AddSub  mode=Subtraction  use_carryin=off  use_carryout=off  en=off  latency=1  precision=User Defined  arith_type="Signed  (2's comp)"  n_bits=2  bin_pt=0  quantization=Truncate  overflow=Saturate  use_behavioral_HDL=off  hw_selection=Fabric  pipelined=off  dbl_ovrd=off  block_type=addsub
  Constant2 : xbsIndex_r4/Constant  const=0  gui_display_data_type=Fixed-point  arith_type=Signed (2's comp)  n_bits=1  bin_pt=0  preci_type=Single  exp_width=8  frac_width=24  explicit_period=off  period=1  equ=P=C  opselect=C  inp2=PCIN>>17  opr=+  inp1=P  carry=CIN  dbl_ovrd=off  block_type=constant
  Constant3 : xbsIndex_r4/Constant  const=0  gui_display_data_type=Fixed-point  arith_type=Signed (2's comp)  n_bits=1  bin_pt=0  preci_type=Single  exp_width=8  frac_width=24  explicit_period=off  period=1  equ=P=C  opselect=C  inp2=PCIN>>17  opr=+  inp1=P  carry=CIN  dbl_ovrd=off  block_type=constant
  Delay4 : xbsIndex_r4/Delay  rst=off  infoeditControl=Selection of Reset will increase slice count due to use of real FFs and instead of SRLs  en=off  latency=1  reg_retiming=off  dbl_ovrd=off  block_type=delay
  Delay5 : xbsIndex_r4/Delay  rst=off  infoeditControl=Selection of Reset will increase slice count due to use of real FFs and instead of SRLs  en=off  latency=1  reg_retiming=off  dbl_ovrd=off  block_type=delay
  Delay6 : xbsIndex_r4/Delay  rst=off  infoeditControl=Selection of Reset will increase slice count due to use of real FFs and instead of SRLs  en=off  latency=1  reg_retiming=off  dbl_ovrd=off  block_type=delay
  Gateway Out{,1..5} (6 alike) : xbsIndex_r4/Gateway Out  inherit_from_input=off  hdl_port=on  rows=1  columns=1  UseAsDAC=off  DACChannel='1'  interface=None  automatic_assignment=on  address_offset=hex2dec('00')  intf_name=''  intf_description=''  timing_constraint=None  locs_specified=off  LOCs={}  io_standard={}  block_type=gatewayout
  Register : xbsIndex_r4/Register  init=0  rst=on  en=on  dbl_ovrd=off  block_type=register
  Register1 : xbsIndex_r4/Register  init=0  rst=on  en=on  dbl_ovrd=off  block_type=register
  Relational : xbsIndex_r4/Relational  mode=a>b  op_type=Bool  en=off  latency=1  dbl_ovrd=off  block_type=relational
  Relational1 : xbsIndex_r4/Relational  mode=a>b  op_type=Bool  en=off  latency=1  dbl_ovrd=off  block_type=relational
  Scope1 : Scope  NumInputPorts=3
  Scope3 : Scope  NumInputPorts=3
  Stop_value : Outport
  Start_value : Outport  Port=2
  wires:
  Gateway Out3/1 -> Scope1/1
  Gateway Out4/1 -> Scope1/2
  Gateway Out5/1 -> Scope1/3
  Gateway Out2/1 -> Scope3/3
  Gateway Out1/1 -> Scope3/2
  Gateway Out/1 -> Scope3/1
  reset/1 -> Register/2, Register1/2, Gateway Out5/1
  window/1 -> Delay6/1, AddSub2/2, Delay4/1, AddSub1/1
  Relational/1 -> Delay5/1
  Register1/1 -> Stop_value/1, Gateway Out4/1
  Relational1/1 -> Register1/3, Gateway Out1/1
  Delay5/1 -> Register/3, Gateway Out2/1
  AddSub1/1 -> Relational/1
  phase/1 -> Register/1, Gateway Out/1, Register1/1
  Delay4/1 -> AddSub1/2
  Delay6/1 -> AddSub2/1
  Constant2/1 -> Relational/2
  AddSub2/1 -> Relational1/1
  Constant3/1 -> Relational1/2
  Register/1 -> Start_value/1, Gateway Out3/1

== system exampleModel_bus_axi_w_4ptavg/example/dsp/Cav1/c1p1_freq_err_module/freq_err1/delta_phi/posedge_pulse ==
  In1 : Inport
  Inverter1 : xbsIndex_r4/Inverter  en=off  latency=20  dbl_ovrd=off  block_type=inv
  Logical : xbsIndex_r4/Logical  logical_function=AND  inputs=2  en=off  latency=1  precision=Full  arith_type=Unsigned  n_bits=16  bin_pt=0  align_bp=on  dbl_ovrd=off  block_type=logical
  Out1 : Outport
  wires:
  Inverter1/1 -> Logical/2
  Logical/1 -> Out1/1
  In1/1 -> Inverter1/1, Logical/1

== system exampleModel_bus_axi_w_4ptavg/example/dsp/Cav1/c1p2_freq_err_module/freq_err1/delta_phi/phase_latching ==
  phase : Inport
  window : Inport  Port=2
  reset : Inport  Port=3
  AddSub1 : xbsIndex_r4/AddSub  mode=Subtraction  use_carryin=off  use_carryout=off  en=off  latency=1  precision=User Defined  arith_type="Signed  (2's comp)"  n_bits=2  bin_pt=0  quantization=Truncate  overflow=Saturate  use_behavioral_HDL=off  hw_selection=Fabric  pipelined=off  dbl_ovrd=off  block_type=addsub
  AddSub2 : xbsIndex_r4/AddSub  mode=Subtraction  use_carryin=off  use_carryout=off  en=off  latency=1  precision=User Defined  arith_type="Signed  (2's comp)"  n_bits=2  bin_pt=0  quantization=Truncate  overflow=Saturate  use_behavioral_HDL=off  hw_selection=Fabric  pipelined=off  dbl_ovrd=off  block_type=addsub
  Constant2 : xbsIndex_r4/Constant  const=0  gui_display_data_type=Fixed-point  arith_type=Signed (2's comp)  n_bits=1  bin_pt=0  preci_type=Single  exp_width=8  frac_width=24  explicit_period=off  period=1  equ=P=C  opselect=C  inp2=PCIN>>17  opr=+  inp1=P  carry=CIN  dbl_ovrd=off  block_type=constant
  Constant3 : xbsIndex_r4/Constant  const=0  gui_display_data_type=Fixed-point  arith_type=Signed (2's comp)  n_bits=1  bin_pt=0  preci_type=Single  exp_width=8  frac_width=24  explicit_period=off  period=1  equ=P=C  opselect=C  inp2=PCIN>>17  opr=+  inp1=P  carry=CIN  dbl_ovrd=off  block_type=constant
  Delay4 : xbsIndex_r4/Delay  rst=off  infoeditControl=Selection of Reset will increase slice count due to use of real FFs and instead of SRLs  en=off  latency=1  reg_retiming=off  dbl_ovrd=off  block_type=delay
  Delay5 : xbsIndex_r4/Delay  rst=off  infoeditControl=Selection of Reset will increase slice count due to use of real FFs and instead of SRLs  en=off  latency=1  reg_retiming=off  dbl_ovrd=off  block_type=delay
  Delay6 : xbsIndex_r4/Delay  rst=off  infoeditControl=Selection of Reset will increase slice count due to use of real FFs and instead of SRLs  en=off  latency=1  reg_retiming=off  dbl_ovrd=off  block_type=delay
  Gateway Out{,1..5} (6 alike) : xbsIndex_r4/Gateway Out  inherit_from_input=off  hdl_port=on  rows=1  columns=1  UseAsDAC=off  DACChannel='1'  interface=None  automatic_assignment=on  address_offset=hex2dec('00')  intf_name=''  intf_description=''  timing_constraint=None  locs_specified=off  LOCs={}  io_standard={}  block_type=gatewayout
  Register : xbsIndex_r4/Register  init=0  rst=on  en=on  dbl_ovrd=off  block_type=register
  Register1 : xbsIndex_r4/Register  init=0  rst=on  en=on  dbl_ovrd=off  block_type=register
  Relational : xbsIndex_r4/Relational  mode=a>b  op_type=Bool  en=off  latency=1  dbl_ovrd=off  block_type=relational
  Relational1 : xbsIndex_r4/Relational  mode=a>b  op_type=Bool  en=off  latency=1  dbl_ovrd=off  block_type=relational
  Scope1 : Scope  NumInputPorts=3
  Scope3 : Scope  NumInputPorts=3
  Stop_value : Outport
  Start_value : Outport  Port=2
  wires:
  Gateway Out3/1 -> Scope1/1
  Gateway Out4/1 -> Scope1/2
  Gateway Out5/1 -> Scope1/3
  Gateway Out2/1 -> Scope3/3
  Gateway Out1/1 -> Scope3/2
  Gateway Out/1 -> Scope3/1
  reset/1 -> Register/2, Register1/2, Gateway Out5/1
  window/1 -> Delay6/1, AddSub2/2, Delay4/1, AddSub1/1
  Relational/1 -> Delay5/1
  Register1/1 -> Stop_value/1, Gateway Out4/1
  Relational1/1 -> Register1/3, Gateway Out1/1
  Delay5/1 -> Register/3, Gateway Out2/1
  AddSub1/1 -> Relational/1
  phase/1 -> Register/1, Gateway Out/1, Register1/1
  Delay4/1 -> AddSub1/2
  Delay6/1 -> AddSub2/1
  Constant2/1 -> Relational/2
  AddSub2/1 -> Relational1/1
  Constant3/1 -> Relational1/2
  Register/1 -> Start_value/1, Gateway Out3/1

== system exampleModel_bus_axi_w_4ptavg/example/dsp/Cav1/c1p2_freq_err_module/freq_err1/delta_phi/posedge_pulse ==
  In1 : Inport
  Inverter1 : xbsIndex_r4/Inverter  en=off  latency=20  dbl_ovrd=off  block_type=inv
  Logical : xbsIndex_r4/Logical  logical_function=AND  inputs=2  en=off  latency=1  precision=Full  arith_type=Unsigned  n_bits=16  bin_pt=0  align_bp=on  dbl_ovrd=off  block_type=logical
  Out1 : Outport
  wires:
  Inverter1/1 -> Logical/2
  Logical/1 -> Out1/1
  In1/1 -> Inverter1/1, Logical/1
